simulink model "Model31"  (R2020a)
settings: Solver=FixedStepDiscrete  StartTime=0.0  StopTime=200  FixedStep=0.1  RelTol=1e-3  EnableMultiTasking=on
settings Model: Creator=HP  LastModifiedBy=HP

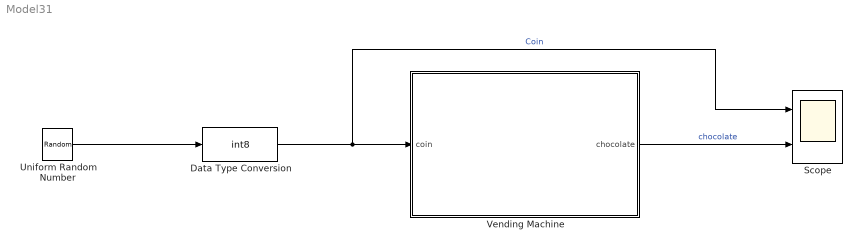
== system Model31 ==
  Data Type Conversion : DataTypeConversion  OutDataTypeStr=int8  RndMeth=Nearest
  Scope : Scope  NumInputPorts=2
  Uniform Random Number : UniformRandomNumber  Minimum=0  Maximum=2  Seed=337  SampleTime=10
  Vending Machine : Stateflow chart  TreatAsAtomicUnit=on
  wires:
  Uniform Random Number/1 -> Data Type Conversion/1
  Data Type Conversion/1 -> Scope/1, Vending Machine/1(coin)  "Coin"
  Vending Machine/1(chocolate) -> Scope/2  "chocolate"

== stateflow chart Model31/Vending Machine ==
  state got_0
  state got_nickel
  state got_dime
  (default) -> got_0
  got_0 -> got_nickel [order 1] : [coin==1]{chocolate=0}
  got_nickel -> got_0 [order 2] : [coin==2]{chocolate=1}
  got_dime -> got_0 [order 1] : [coin==1]{chocolate=1}
  got_0 -> got_dime [order 2] : [coin==2]{chocolate=0}
  got_nickel -> got_dime [order 1] : [coin==1]{chocolate=0}
  got_dime -> got_nickel [order 2] : [coin==2]{chocolate=1}
  data: coin input; chocolate output
